simulink model "Proxy_based_Sliding_mode_control_Crane"  (R2019a)
settings: Solver=ode1  StartTime=0.0  StopTime=20  FixedStep=0.01  RelTol=1e-3
InitFcn:
  | M =1.155+2.20;
  | m = 1;
  | Dx  =0.5;
  | L = 0.5;
  | g = 9.8;
undefined symbols (not defined in the file or in its folder): magnitude
settings Model: Creator=pablo.prieto  LastModifiedBy=dell
settings DataIOCC: SaveFormat=StructureWithTime  ReturnWorkspaceOutputs=off
settings OptimizationCC: LifeSpan=inf
settings DebuggingCC: ArithmeticOperatorsInVariantConditions=warning
settings HardwareCC: ProdBitPerSizeT=32  ProdBitPerPtrDiffT=32  ProdWordSize=32  ProdHWDeviceType=Specified
settings SFSimCC: SimUseLocalCustomCode=off
settings RTWCC: RTWUseLocalCustomCode=off
settings CodeAppCC: StateflowObjectComments=on
settings GRTTargetCC: TargetLangStandard=C89/C90 (ANSI)

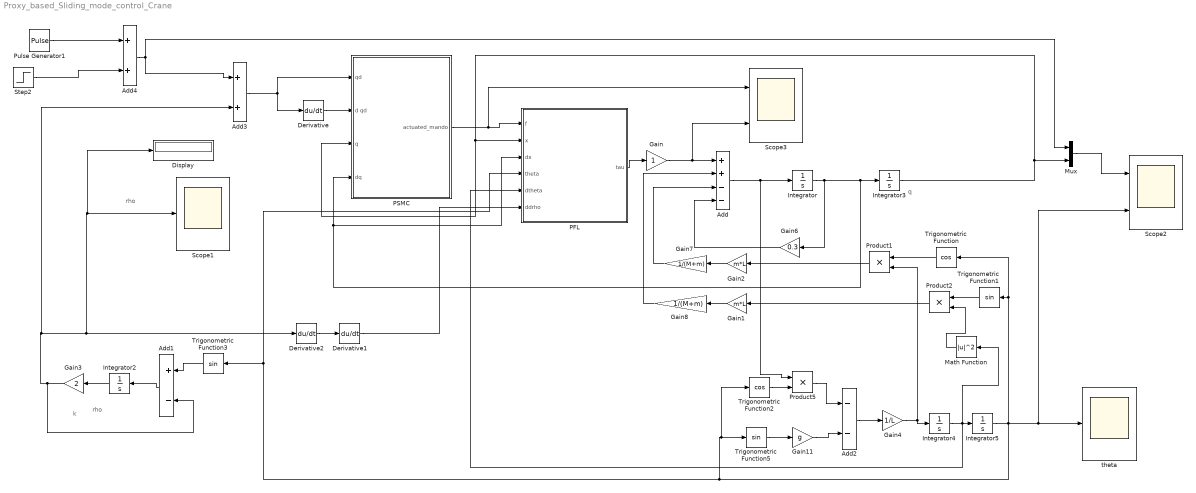
== system Proxy_based_Sliding_mode_control_Crane ==
  note: q
  note: rho
  note: rho
  note: k
  Add : Sum  Inputs=++--
  Add1 : Sum  Inputs=+-
  Add2 : Sum  Inputs=--
  Add3 : Sum
  Add4 : Sum
  Derivative : Derivative
  Derivative1 : Derivative
  Derivative2 : Derivative
  Display : Display
  Gain : Gain
  Gain1 : Gain  Gain=m*L
  Gain11 : Gain  Gain=g
  Gain2 : Gain  Gain=m*L
  Gain3 : Gain  Gain=2
  Gain4 : Gain  Gain=1/L
  Gain6 : Gain  Gain=0.3
  Gain7 : Gain  Gain=1/(M+m)
  Gain8 : Gain  Gain=1/(M+m)
  Integrator{,2..5} (5 alike) : Integrator
  Math Function : Math  Operator=magnitude^2  SaturateOnIntegerOverflow=on
  Mux : Mux  Inputs=2
  PFL : MATLAB Function  TreatAsAtomicUnit=on
  PSMC : Subsystem  mask{H=1.5, K=30, B=25, F=1}
      mask prompts: H "Constant Time(H)"; K "Proportional Gain(K)"; B "Derivative Gain(B)"; F "Robust Gain(F)"
  Product1 : Product
  Product2 : Product
  Product5 : Product
  Pulse Generator1 : DiscretePulseGenerator  PulseType=Time based  Amplitude=0.4  Period=40  PulseWidth=50
  Scope1 : Scope
  Scope2 : Scope  NumInputPorts=2
  Scope3 : Scope  NumInputPorts=2
  Step2 : Step  Time=20  After=0.1  SampleTime=0
  Trigonometric Function : Trigonometry  Operator=cos
  Trigonometric Function1 : Trigonometry
  Trigonometric Function2 : Trigonometry  Operator=cos
  Trigonometric Function3 : Trigonometry
  Trigonometric Function5 : Trigonometry
  theta : Scope
  wires:
  Add/1 -> Product5/1, Integrator/1
  Integrator/1 -> Gain6/1, PFL/3(dx), PSMC/4(dq), Integrator3/1
  Gain2/1 -> Gain7/1
  Gain1/1 -> Gain8/1
  Trigonometric Function/1 -> Product1/1
  Product1/1 -> Gain2/1
  Gain11/1 -> Add2/2
  Product5/1 -> Add2/1
  Trigonometric Function5/1 -> Gain11/1
  Trigonometric Function2/1 -> Product5/2
  Add2/1 -> Gain4/1
  Integrator4/1 -> PFL/5(dtheta), Math Function/1, Integrator5/1
  Trigonometric Function1/1 -> Product2/1
  Product2/1 -> Gain1/1
  Math Function/1 -> Product2/2
  Integrator3/1 -> Mux/2, PFL/2(x), PSMC/3(q)
  Mux/1 -> Scope2/1
  Derivative/1 -> PSMC/2(d qd)
  Gain7/1 -> Add/3
  Gain8/1 -> Add/2
  PFL/1(tau) -> Gain/1
  Gain6/1 -> Add/4
  Derivative1/1 -> PFL/6(ddrho)
  Derivative2/1 -> Derivative1/1
  Pulse Generator1/1 -> Add4/1
  Step2/1 -> Add4/2
  Gain4/1 -> Integrator4/1, Product1/2
  PSMC/1(actuated_mando) -> Scope3/1, PFL/1(f)
  Integrator2/1 -> Gain3/1
  Integrator5/1 -> Trigonometric Function3/1, PFL/4(theta), Trigonometric Function2/1, Trigonometric Function5/1, theta/1, Scope2/2, Trigonometric Function1/1, Trigonometric Function/1
  Trigonometric Function3/1 -> Add1/1
  Gain3/1 -> Add1/2, Add3/2, Derivative2/1, Display/1, Scope1/1
  Add1/1 -> Integrator2/1
  Add3/1 -> Derivative/1, PSMC/1(qd)
  Add4/1 -> Add3/1, Mux/1
  Gain/1 -> Scope3/2, Add/1

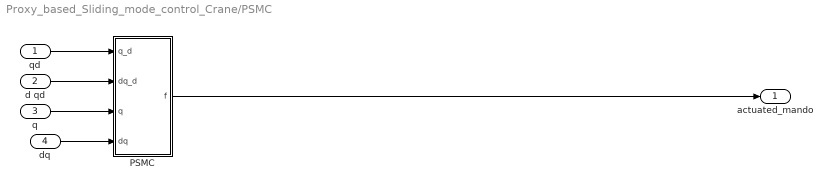
== system Proxy_based_Sliding_mode_control_Crane/PSMC ==
  qd : Inport
  d qd : Inport  Port=2
  q : Inport  Port=3
  dq : Inport  Port=4
  PSMC : Subsystem
  actuated_mando : Outport
  wires:
  d qd/1 -> PSMC/2(dq_d)
  qd/1 -> PSMC/1("q_d ")
  dq/1 -> PSMC/4(dq)
  q/1 -> PSMC/3(q)
  PSMC/1(f) -> actuated_mando/1

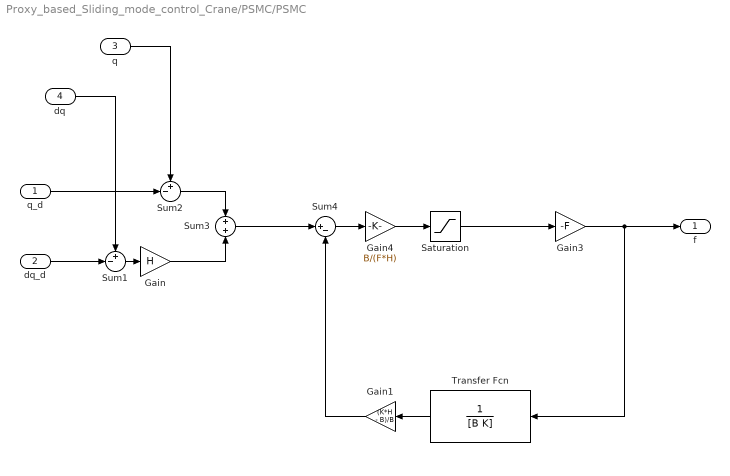
== system Proxy_based_Sliding_mode_control_Crane/PSMC/PSMC ==
  "q_d " : Inport
  dq_d : Inport  Port=2
  q : Inport  Port=3
  dq : Inport  Port=4
  Gain : Gain  Gain=H
  Gain1 : Gain  Gain=(K*H - B)/B
  Gain3 : Gain  Gain=-F
  Gain4 : Gain  Gain=B/(F*H)
  Saturation : Saturate  UpperLimit=1  LowerLimit=-1
  Sum1 : Sum  Inputs=+-|
  Sum2 : Sum  Inputs=+-|
  Sum3 : Sum
  Sum4 : Sum  Inputs=|+-
  Transfer Fcn : TransferFcn  Numerator=1  Denominator=[B K]
  f : Outport
  wires:
  Sum2/1 -> Sum3/1
  q/1 -> Sum2/1
  "q_d "/1 -> Sum2/2
  dq/1 -> Sum1/1
  dq_d/1 -> Sum1/2
  Sum1/1 -> Gain/1
  Gain/1 -> Sum3/2
  Sum4/1 -> Gain4/1
  Saturation/1 -> Gain3/1
  Sum3/1 -> Sum4/1
  Gain3/1 -> Transfer Fcn/1, f/1
  Gain1/1 -> Sum4/2
  Transfer Fcn/1 -> Gain1/1
  Gain4/1 -> Saturation/1

== matlab function Proxy_based_Sliding_mode_control_Crane/PFL ==
  data: f input; x input; dx input; theta input; dtheta input; tau output; ddrho input
function tau = fcn(f,x,dx,theta,dtheta,ddrho)

g=9.81;
Mx = 1.155+2.20;
m = 1;
L = 0.5;

%parámetros de M
m11 = m*L^2;
m12 = m*L*cos(theta);
m21 = m12;
m22 = Mx + m;

Dq = 0.3;

h2 = -m*L*sin(theta)*dtheta^2;





tau = (m22-m*cos(theta)^2)*(ddrho+f)-m*g*sin(2*theta)/2+h2+ Dq*dx;
